simulink model "Drone2"  (R2020a)
settings: Solver=VariableStepAuto  StartTime=0.0  StopTime=20  RelTol=1e-3
values from neighbouring files (symbols this model uses):
  b = 1.84E-7    (= 1.84e-07)    [DroneControlPID.m]    (also in Drone_Control4.m = 1.98e-07; Drone_Control5.m = 1.98e-07)
  Ixx = 0.0118    [DroneControlPID.m]    (also in Drone_Control4.m = 0.0116; Drone_Control5.m = 0.0116)
  Iyy = 0.0118    [DroneControlPID.m]    (also in Drone_Control4.m = 0.0225; Drone_Control5.m = 0.0225)
  Izz = 0.0225    [DroneControlPID.m]    (also in Drone_Control4.m = 0.0121; Drone_Control5.m = 0.0121)
  k = 3.24E-8    (= 3.24e-08)    [DroneControlPID.m]    (also in Drone_Control4.m = 7.78e-06; Drone_Control5.m = 7.78e-06)
  L = 0.225    [DroneControlPID.m]    (also in Drone_Control4.m = 160; Drone_Control5.m = 0.16)
  Ts = 0.007    [DroneControlPID.m]    (also in Drone_Control5.m = 0.07)
settings Model: Creator=Evans  LastModifiedBy=Evans

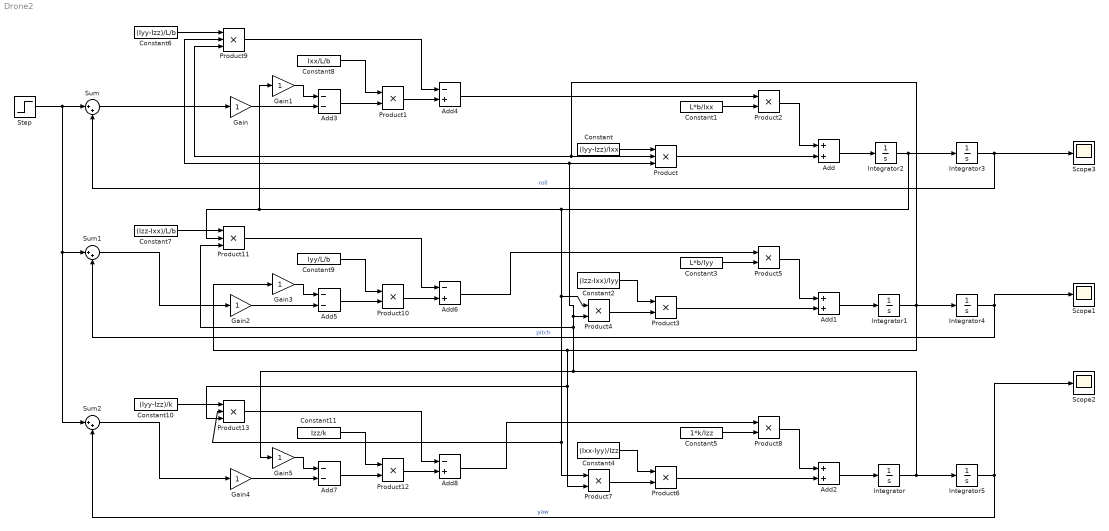
== system Drone2 ==
  Add : Sum
  Add1 : Sum
  Add2 : Sum
  Add3 : Sum  Inputs=--
  Add4 : Sum  Inputs=-+
  Add5 : Sum  Inputs=--
  Add6 : Sum  Inputs=-+
  Add7 : Sum  Inputs=--
  Add8 : Sum  Inputs=-+
  Constant : Constant  Value=(Iyy-Izz)/Ixx  SampleTime=Ts
  Constant1 : Constant  Value=L*b/Ixx  SampleTime=Ts
  Constant10 : Constant  Value=(Iyy-Izz)/k  SampleTime=Ts
  Constant11 : Constant  Value=Izz/k  SampleTime=Ts
  Constant2 : Constant  Value=(Izz-Ixx)/Iyy  SampleTime=Ts
  Constant3 : Constant  Value=L*b/Iyy  SampleTime=Ts
  Constant4 : Constant  Value=(Ixx-Iyy)/Izz  SampleTime=Ts
  Constant5 : Constant  Value=1*k/Izz  SampleTime=Ts
  Constant6 : Constant  Value=(Iyy-Izz)/L/b  SampleTime=Ts
  Constant7 : Constant  Value=(Izz-Ixx)/L/b  SampleTime=Ts
  Constant8 : Constant  Value=Ixx/L/b  SampleTime=Ts
  Constant9 : Constant  Value=Iyy/L/b  SampleTime=Ts
  Gain{,1..5} (6 alike) : Gain
  Integrator : Integrator
  Integrator1 : Integrator
  Integrator2 : Integrator
  Integrator3 : Integrator  InitialCondition=1
  Integrator4 : Integrator  InitialCondition=1
  Integrator5 : Integrator  InitialCondition=1
  Product{,9,11,13} (4 alike) : Product  Inputs=3
  Product{1..8,10,12} (10 alike) : Product
  Scope1 : Scope
  Scope2 : Scope
  Scope3 : Scope
  Step : Step  Time=0  After=0  SampleTime=Ts
  Sum : Sum  Inputs=|++
  Sum1 : Sum  Inputs=|++
  Sum2 : Sum  Inputs=|++
  wires:
  Integrator3/1 -> Scope3/1, Sum/2  "roll"
  Integrator4/1 -> Sum1/2, Scope1/1  "pitch"
  Integrator5/1 -> Scope2/1, Sum2/2  "yaw"
  Step/1 -> Sum2/1, Sum1/1, Sum/1
  Constant3/1 -> Product5/2
  Constant4/1 -> Product6/1
  Product6/1 -> Add2/2
  Integrator1/1 -> Product9/3, Product/2, Integrator4/1, Gain3/1, Product7/2, Product13/3
  Add2/1 -> Integrator/1
  Integrator/1 -> Integrator5/1, Gain5/1, Product9/2, Product/3, Product4/2, Product11/3
  Product7/1 -> Product6/2
  Add/1 -> Integrator2/1
  Add1/1 -> Integrator1/1
  Constant5/1 -> Product8/2
  Product2/1 -> Add/1
  Constant1/1 -> Product2/2
  Product5/1 -> Add1/1
  Product/1 -> Add/2
  Constant/1 -> Product/1
  Product4/1 -> Product3/2
  Product3/1 -> Add1/2
  Constant2/1 -> Product3/1
  Product8/1 -> Add2/1
  Constant6/1 -> Product9/1
  Sum/1 -> Gain/1
  Integrator2/1 -> Product11/2, Gain1/1, Product13/2, Product7/1, Product4/1, Integrator3/1
  Gain1/1 -> Add3/1
  Gain/1 -> Add3/2
  Constant8/1 -> Product1/1
  Add3/1 -> Product1/2
  Product1/1 -> Add4/2
  Product9/1 -> Add4/1
  Add4/1 -> Product2/1
  Product10/1 -> Add6/2
  Gain3/1 -> Add5/1
  Add5/1 -> Product10/2
  Gain2/1 -> Add5/2
  Product11/1 -> Add6/1
  Constant9/1 -> Product10/1
  Constant7/1 -> Product11/1
  Gain5/1 -> Add7/1
  Add7/1 -> Product12/2
  Constant11/1 -> Product12/1
  Product13/1 -> Add8/1
  Constant10/1 -> Product13/1
  Gain4/1 -> Add7/2
  Product12/1 -> Add8/2
  Add6/1 -> Product5/1
  Add8/1 -> Product8/1
  Sum1/1 -> Gain2/1
  Sum2/1 -> Gain4/1
